simulink model "RIFDSimulink"  (R2016a)
settings: Solver=FixedStepAuto  StartTime=0.0  StopTime=0.0123  RelTol=1e-3
values from neighbouring files (symbols this model uses):
  b1 = fir1(fir_order, freq2rad(filters_freqs, fs), 'bandpass', ones(fir_order+1, 1))    [bandpass_test.m]
  fs = 4224000    [bandpass_test.m]    (also in graphs.m = 50688000; main.m = 2*max_stop_freq_fir; rf_controller.m = 1/(time(2)-time(1)))
undefined symbols (not defined in the file or in its folder): b2, b_fir_kaiser, baud, DelayLengthBandPass, DelayLengthLowPass, Sigma
libraries: dspsigops x6, simulink x2
settings Model: Creator=spip2401  LastModifiedBy=spip2401

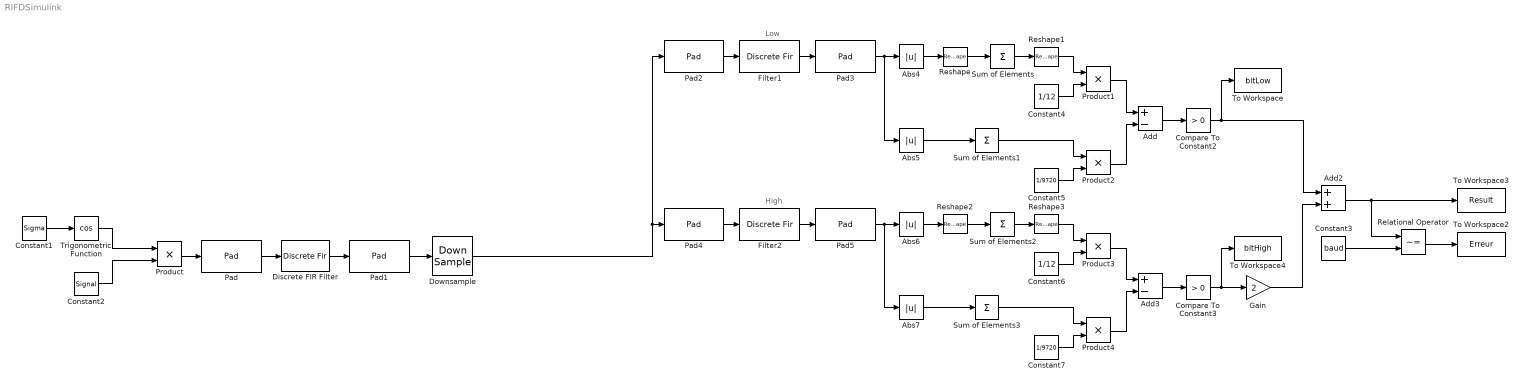
== system RIFDSimulink ==
  note: Low
  note: High
  Abs{4..7} (4 alike) : Abs
  Add : Sum  Inputs=+-
  Add2 : Sum
  Add3 : Sum  Inputs=+-
  Compare To Constant2 : simulink/Logic and Bit Operations/Compare To Constant  relop=>  const=0  OutDataTypeStr=boolean
  Compare To Constant3 : simulink/Logic and Bit Operations/Compare To Constant  relop=>  const=0  OutDataTypeStr=boolean
  Constant1 : Constant  Value=Sigma  SampleTime=fs
  Constant2 : Constant  Value=Signal  SampleTime=fs
  Constant3 : Constant  Value=baud  SampleTime=fs
  Constant4 : Constant  Value=1/12  SampleTime=fs
  Constant5 : Constant  Value=1/9720  SampleTime=fs
  Constant6 : Constant  Value=1/12  SampleTime=fs
  Constant7 : Constant  Value=1/9720  SampleTime=fs
  Discrete FIR Filter : DiscreteFir  Coefficients=b_fir_kaiser  InputProcessing=Columns as channels (frame based)
  Downsample : DownSample  N=64
  Filter1 : DiscreteFir  Tag=BlockMethodSubSystem  Coefficients=b1  InputProcessing=Columns as channels (frame based)
  Filter2 : DiscreteFir  Tag=BlockMethodSubSystem  Coefficients=b2  InputProcessing=Columns as channels (frame based)
  Gain : Gain  Gain=2
  Pad : dspsigops/Pad  padAlong=Columns  dimsToPad=1  valSrc=Specify via dialog  padVal=0  spec=Output size  padNumOutRowsSpecMethod=User-specified  numOutRows=DelayLengthLowPass+10  padNumOutColsSpecMethod=User-specified  numOutCols=1  isVarDimsMode=off  padBeginning=0  padEnd=0  outSizeMode=User-specified  outSize=1  padSigAt=End  trunc_flag=None  roundingMode=Floor  overflowMode=off  truncOrWrapMode=Truncate  wrap_flag=None
  Pad1 : dspsigops/Pad  padAlong=Columns  dimsToPad=1  valSrc=Specify via dialog  padVal=0  spec=Output size  padNumOutRowsSpecMethod=User-specified  numOutRows=DelayLengthLowPass  padNumOutColsSpecMethod=User-specified  numOutCols=1  isVarDimsMode=off  padBeginning=0  padEnd=0  outSizeMode=User-specified  outSize=1  padSigAt=Beginning  trunc_flag=None  roundingMode=Floor  overflowMode=off  truncOrWrapMode=Truncate  wrap_flag=None
  Pad2 : dspsigops/Pad  padAlong=Columns  dimsToPad=1  valSrc=Specify via dialog  padVal=0  spec=Output size  padNumOutRowsSpecMethod=User-specified  numOutRows=DelayLengthBandPass+25  padNumOutColsSpecMethod=User-specified  numOutCols=1  isVarDimsMode=off  padBeginning=0  padEnd=0  outSizeMode=User-specified  outSize=1  padSigAt=End  trunc_flag=None  roundingMode=Floor  overflowMode=off  truncOrWrapMode=Truncate  wrap_flag=None
  Pad3 : dspsigops/Pad  padAlong=Columns  dimsToPad=1  valSrc=Specify via dialog  padVal=0  spec=Output size  padNumOutRowsSpecMethod=User-specified  numOutRows=DelayLengthBandPass  padNumOutColsSpecMethod=User-specified  numOutCols=1  isVarDimsMode=off  padBeginning=0  padEnd=0  outSizeMode=User-specified  outSize=1  padSigAt=Beginning  trunc_flag=None  roundingMode=Floor  overflowMode=off  truncOrWrapMode=Truncate  wrap_flag=None
  Pad4 : dspsigops/Pad  padAlong=Columns  dimsToPad=1  valSrc=Specify via dialog  padVal=0  spec=Output size  padNumOutRowsSpecMethod=User-specified  numOutRows=DelayLengthBandPass+25  padNumOutColsSpecMethod=User-specified  numOutCols=1  isVarDimsMode=off  padBeginning=0  padEnd=0  outSizeMode=User-specified  outSize=1  padSigAt=End  trunc_flag=None  roundingMode=Floor  overflowMode=off  truncOrWrapMode=Truncate  wrap_flag=None
  Pad5 : dspsigops/Pad  padAlong=Columns  dimsToPad=1  valSrc=Specify via dialog  padVal=0  spec=Output size  padNumOutRowsSpecMethod=User-specified  numOutRows=DelayLengthBandPass  padNumOutColsSpecMethod=User-specified  numOutCols=1  isVarDimsMode=off  padBeginning=0  padEnd=0  outSizeMode=User-specified  outSize=1  padSigAt=Beginning  trunc_flag=None  roundingMode=Floor  overflowMode=off  truncOrWrapMode=Truncate  wrap_flag=None
  Product{,1..4} (5 alike) : Product
  Relational Operator : RelationalOperator  Operator=~=  OutDataTypeStr=boolean
  Reshape : Reshape  OutputDimensionality=Customize  OutputDimensions=[12,810]
  Reshape1 : Reshape  OutputDimensionality=Column vector (2-D)  OutputDimensions=[810,1]
  Reshape2 : Reshape  OutputDimensionality=Customize  OutputDimensions=[12,810]
  Reshape3 : Reshape  OutputDimensionality=Column vector (2-D)  OutputDimensions=[810,1]
  Sum of Elements{,1..3} (4 alike) : Sum  Inputs=+  CollapseMode=Specified dimension
  To Workspace : ToWorkspace  VariableName=bitLow  SampleTime=-1
      settings: Save2DSignal=2-D array (concatenate along first dimension)
  To Workspace2 : ToWorkspace  VariableName=Erreur  SampleTime=-1
      settings: Save2DSignal=2-D array (concatenate along first dimension)
  To Workspace3 : ToWorkspace  VariableName=Result  SampleTime=-1
      settings: Save2DSignal=2-D array (concatenate along first dimension)
  To Workspace4 : ToWorkspace  VariableName=bitHigh  SampleTime=-1
      settings: Save2DSignal=2-D array (concatenate along first dimension)
  Trigonometric Function : Trigonometry  Operator=cos
  wires:
  Constant1/1 -> Trigonometric Function/1
  Trigonometric Function/1 -> Product/1
  Constant2/1 -> Product/2
  Product/1 -> Pad/1
  Add2/1 -> To Workspace3/1, Relational Operator/1
  Constant3/1 -> Relational Operator/2
  Relational Operator/1 -> To Workspace2/1
  Compare To Constant2/1 -> Add2/1, To Workspace/1
  Filter1/1 -> Pad3/1
  Sum of Elements/1 -> Reshape1/1
  Constant4/1 -> Product1/2
  Abs4/1 -> Reshape/1
  Reshape/1 -> Sum of Elements/1
  Reshape1/1 -> Product1/1
  Product1/1 -> Add/1
  Constant5/1 -> Product2/2
  Abs5/1 -> Sum of Elements1/1
  Product2/1 -> Add/2
  Sum of Elements1/1 -> Product2/1
  Add/1 -> Compare To Constant2/1
  Pad/1 -> Discrete FIR Filter/1
  Pad2/1 -> Filter1/1
  Pad3/1 -> Abs5/1, Abs4/1
  Discrete FIR Filter/1 -> Pad1/1
  Pad1/1 -> Downsample/1
  Filter2/1 -> Pad5/1
  Sum of Elements2/1 -> Reshape3/1
  Constant6/1 -> Product3/2
  Abs6/1 -> Reshape2/1
  Reshape2/1 -> Sum of Elements2/1
  Reshape3/1 -> Product3/1
  Product3/1 -> Add3/1
  Constant7/1 -> Product4/2
  Abs7/1 -> Sum of Elements3/1
  Product4/1 -> Add3/2
  Sum of Elements3/1 -> Product4/1
  Add3/1 -> Compare To Constant3/1
  Pad4/1 -> Filter2/1
  Pad5/1 -> Abs7/1, Abs6/1
  Compare To Constant3/1 -> Gain/1, To Workspace4/1
  Gain/1 -> Add2/2
  Downsample/1 -> Pad2/1, Pad4/1
